simulink model "Ex2_2"  (R2016a)
settings: Solver=VariableStepAuto  StartTime=0.0  StopTime=2  RelTol=1e-3
settings Model: Creator=mende  LastModifiedBy=mende

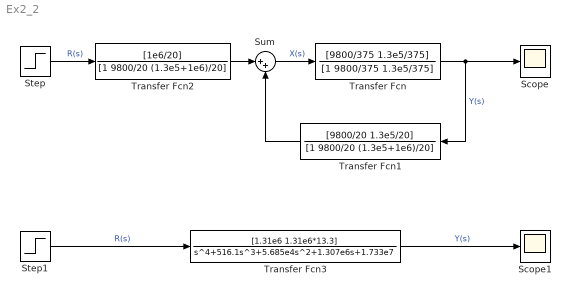
== system Ex2_2 ==
  Scope : Scope
  Scope1 : Scope
  Step : Step  SampleTime=0
  Step1 : Step  SampleTime=0
  Sum : Sum  Inputs=|++
  Transfer Fcn : TransferFcn  Numerator=[9800/375 1.3e5/375]  Denominator=[1 9800/375 1.3e5/375]
  Transfer Fcn1 : TransferFcn  Numerator=[9800/20 1.3e5/20]  Denominator=[1 9800/20 (1.3e5+1e6)/20]
  Transfer Fcn2 : TransferFcn  Numerator=[1e6/20]  Denominator=[1 9800/20 (1.3e5+1e6)/20]
  Transfer Fcn3 : TransferFcn  Numerator=[1.31e6 1.31e6*13.3]  Denominator=[1 516.1 5.685e4 1.307e6 1.733e7]
  wires:
  Sum/1 -> Transfer Fcn/1  "X(s)"
  Transfer Fcn1/1 -> Sum/2
  Transfer Fcn/1 -> Scope/1, Transfer Fcn1/1  "Y(s)"
  Transfer Fcn2/1 -> Sum/1
  Step/1 -> Transfer Fcn2/1  "R(s)"
  Transfer Fcn3/1 -> Scope1/1  "Y(s)"
  Step1/1 -> Transfer Fcn3/1  "R(s)"
